simulink model "Class_exp1"  (R2024b)
settings: Solver=FixedStepAuto  StartTime=0.0  StopTime=1.0  FixedStep=1e-6  RelTol=1e-4  AbsTol=1e-5
libraries: simulink x1
settings Model: Creator=86195  LastModifiedBy=86195

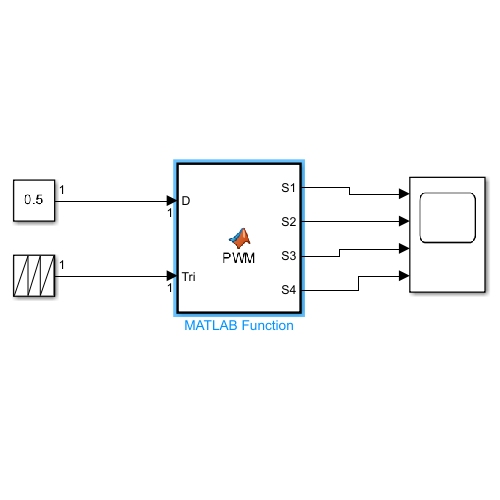
[thumbnail: Simulink's stored preview of the top-level diagram]
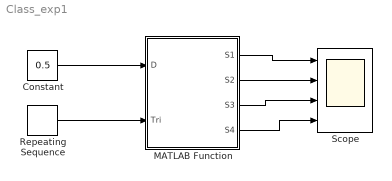
== system Class_exp1 ==
  Constant : Constant  Value=0.5
  MATLAB Function : MATLAB Function  TreatAsAtomicUnit=on
  Repeating Sequence : simulink/Sources/Repeating Sequence  rep_seq_t=[0 1e-4]  rep_seq_y=[0 1]
  Scope : Scope  NumInputPorts=4
  wires:
  Constant/1 -> MATLAB Function/1(D)
  Repeating Sequence/1 -> MATLAB Function/2(Tri)
  MATLAB Function/1(S1) -> Scope/1
  MATLAB Function/2(S2) -> Scope/2
  MATLAB Function/3(S3) -> Scope/3
  MATLAB Function/4(S4) -> Scope/4

== matlab function Class_exp1/MATLAB Function ==
  data: D input; S1 output; Tri input; S2 output; S3 output; S4 output
function [S1,S2,S3,S4] = PWM(D,Tri)

if (D >= Tri)
        S1 = 1;
else
        S1 = 0;
end

if (Tri >= 0.1)&&(Tri <= D+0.1)
        S3 = 1;
else
        S3 = 0;
end

S4 = 1 - S3;
S2 = 1 - S1;
